simulink model "Laptrinhquydao"  (R2020a)
settings: Solver=VariableStepAuto  StartTime=0.0  StopTime=10.0  RelTol=1e-3
settings Model: Creator=dell  LastModifiedBy=dell

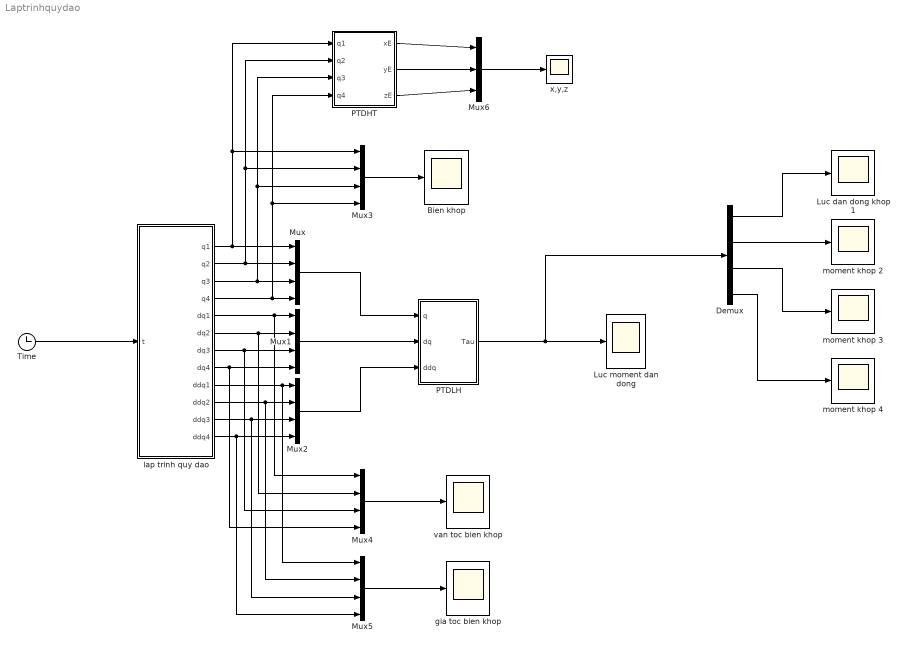
== system Laptrinhquydao ==
  Bien khop : Scope
  Demux : Demux
  "Luc dan dong khop 1 " : Scope
  Luc moment dan dong : Scope
  Mux{,1..5} (6 alike) : Mux
  Mux6 : Mux  Inputs=3
  PTDHT : MATLAB Function  TreatAsAtomicUnit=on
  PTDLH : MATLAB Function  TreatAsAtomicUnit=on
  "Time " : Clock
  gia toc bien khop : Scope
  lap trinh quy dao : MATLAB Function  TreatAsAtomicUnit=on
  moment khop 2 : Scope
  moment khop 3 : Scope
  moment khop 4 : Scope
  "van toc bien khop " : Scope
  x,y,z : Scope
  wires:
  "Time "/1 -> lap trinh quy dao/1(t)
  lap trinh quy dao/1(q1) -> Mux3/1, PTDHT/1(q1), Mux/1
  lap trinh quy dao/2(q2) -> Mux3/2, PTDHT/2(q2), Mux/2
  lap trinh quy dao/3(q3) -> Mux3/3, PTDHT/3(q3), Mux/3
  lap trinh quy dao/4(q4) -> Mux3/4, PTDHT/4(q4), Mux/4
  lap trinh quy dao/5(dq1) -> Mux4/1, Mux1/1
  lap trinh quy dao/6(dq2) -> Mux4/2, Mux1/2
  lap trinh quy dao/7(dq3) -> Mux4/3, Mux1/3
  lap trinh quy dao/8(dq4) -> Mux4/4, Mux1/4
  lap trinh quy dao/9(ddq1) -> Mux5/1, Mux2/1
  lap trinh quy dao/10(ddq2) -> Mux5/2, Mux2/2
  lap trinh quy dao/11(ddq3) -> Mux5/3, Mux2/3
  lap trinh quy dao/12(ddq4) -> Mux5/4, Mux2/4
  Mux1/1 -> PTDLH/2(dq)
  Mux/1 -> PTDLH/1(q)
  Mux2/1 -> PTDLH/3(ddq)
  PTDLH/1(Tau) -> Demux/1, Luc moment dan dong/1
  Mux3/1 -> Bien khop/1
  Mux4/1 -> "van toc bien khop "/1
  Mux5/1 -> gia toc bien khop/1
  Demux/1 -> "Luc dan dong khop 1 "/1
  Demux/2 -> moment khop 2/1
  Demux/3 -> moment khop 3/1
  Demux/4 -> moment khop 4/1
  PTDHT/2(yE) -> Mux6/2
  PTDHT/1(xE) -> Mux6/1
  PTDHT/3(zE) -> Mux6/3
  Mux6/1 -> x,y,z/1

== matlab function Laptrinhquydao/PTDLH ==
  data: q input; Tau output; dq input; ddq input
function Tau = fcn(q,dq,ddq)

[L1, L2, L3, L4,L0,m1,m2,m3,m4,I1x,I1y,I1z,I2x,I2y,I2z,I3x,I3y,I3z,I4x,I4y,I4z]=Parameters();

M=zeros(4,4);
M(1,1)= m1 + m2 + m3 + m4;
M(1,2)= ((-0.3e1 * m4 * L4 * cos(q(4)) - 0.3e1 * L3 * (m3 + 0.2e1 / 0.3e1 * m4)) * cos(q(3)) + 0.3e1 * sin(q(3)) * sin(q(4)) * L4 * m4 - 0.3e1 * L2 * (m2 + 0.2e1 / 0.3e1 * m3 + 0.2e1 / 0.3e1 * m4)) * cos(q(2)) / 0.2e1 + 0.3e1 / 0.2e1 * sin(q(2)) * (sin(q(4)) * L4 * m4 * cos(q(3)) + (m4 * L4 * cos(q(4)) + L3 * (m3 + 0.2e1 / 0.3e1 * m4)) * sin(q(3)));
M(1,3)= ((-0.3e1 * m4 * L4 * cos(q(4)) - 0.3e1 * L3 * (m3 + 0.2e1 / 0.3e1 * m4)) * cos(q(3)) + 0.3e1 * sin(q(3)) * sin(q(4)) * L4 * m4) * cos(q(2)) / 0.2e1 + 0.3e1 / 0.2e1 * sin(q(2)) * (sin(q(4)) * L4 * m4 * cos(q(3)) + (m4 * L4 * cos(q(4)) + L3 * (m3 + 0.2e1 / 0.3e1 * m4)) * sin(q(3)));
M(1,4)= 0.3e1 / 0.2e1 * L4 * ((sin(q(2)) * sin(q(3)) - cos(q(2)) * cos(q(3))) * cos(q(4)) + sin(q(4)) * (cos(q(2)) * sin(q(3)) + sin(q(2)) * cos(q(3)))) * m4;

M(2,1)= ((-0.3e1 * m4 * L4 * cos(q(4)) - 0.3e1 * L3 * (m3 + 0.2e1 / 0.3e1 * m4)) * cos(q(3)) + 0.3e1 * sin(q(3)) * sin(q(4)) * L4 * m4 - 0.3e1 * L2 * (m2 + 0.2e1 / 0.3e1 * m3 + 0.2e1 / 0.3e1 * m4)) * cos(q(2)) / 0.2e1 + 0.3e1 / 0.2e1 * sin(q(2)) * (sin(q(4)) * L4 * m4 * cos(q(3)) + (m4 * L4 * cos(q(4)) + L3 * (m3 + 0.2e1 / 0.3e1 * m4)) * sin(q(3)));
M(2,2)= 0.3e1 * L2 * (m4 * L4 * cos(q(4)) + L3 * (m3 + 0.2e1 / 0.3e1 * m4)) * cos(q(3)) + 0.3e1 * m4 * L4 * L3 * cos(q(4)) - 0.3e1 * m4 * L4 * L2 * sin(q(4)) * sin(q(3)) + ((9 * m2) + 0.4e1 * m3 + 0.4e1 * m4) * L2 ^ 2 / 0.4e1 + (0.4e1 * L3 ^ 2 + 0.9e1 * L4 ^ 2) * m4 / 0.4e1 + 0.9e1 / 0.4e1 * m3 * L3 ^ 2 + I3z + I4z + I2z;
M(2,3)= 0.3e1 / 0.2e1 * L2 * (m4 * L4 * cos(q(4)) + L3 * (m3 + 0.2e1 / 0.3e1 * m4)) * cos(q(3)) + 0.3e1 * m4 * L4 * L3 * cos(q(4)) - 0.3e1 / 0.2e1 * m4 * L4 * L2 * sin(q(4)) * sin(q(3)) + (0.4e1 * L3 ^ 2 + 0.9e1 * L4 ^ 2) * m4 / 0.4e1 + 0.9e1 / 0.4e1 * m3 * L3 ^ 2 + I3z + I4z;
M(2,4)= 0.3e1 / 0.2e1 * m4 * L4 * (L2 * cos(q(3)) + L3) * cos(q(4)) - 0.3e1 / 0.2e1 * m4 * L4 * L2 * sin(q(4)) * sin(q(3)) + 0.9e1 / 0.4e1 * m4 * L4 ^ 2 + I4z;

M(3,1)= ((-0.3e1 * m4 * L4 * cos(q(4)) - 0.3e1 * L3 * (m3 + 0.2e1 / 0.3e1 * m4)) * cos(q(3)) + 0.3e1 * sin(q(3)) * sin(q(4)) * L4 * m4) * cos(q(2)) / 0.2e1 + 0.3e1 / 0.2e1 * sin(q(2)) * (sin(q(4)) * L4 * m4 * cos(q(3)) + (m4 * L4 * cos(q(4)) + L3 * (m3 + 0.2e1 / 0.3e1 * m4)) * sin(q(3)));
M(3,2)= 0.3e1 / 0.2e1 * L2 * (m4 * L4 * cos(q(4)) + L3 * (m3 + 0.2e1 / 0.3e1 * m4)) * cos(q(3)) + 0.3e1 * m4 * L4 * L3 * cos(q(4)) - 0.3e1 / 0.2e1 * m4 * L4 * L2 * sin(q(4)) * sin(q(3)) + (0.4e1 * L3 ^ 2 + 0.9e1 * L4 ^ 2) * m4 / 0.4e1 + 0.9e1 / 0.4e1 * m3 * L3 ^ 2 + I3z + I4z;
M(3,3)= 0.3e1 * m4 * L4 * L3 * cos(q(4)) + ((9 * m3) + 0.4e1 * m4) * L3 ^ 2 / 0.4e1 + 0.9e1 / 0.4e1 * m4 * L4 ^ 2 + I3z + I4z;
M(3,4)= 0.3e1 / 0.2e1 * m4 * L4 * L3 * cos(q(4)) + 0.9e1 / 0.4e1 * m4 * L4 ^ 2 + I4z;

M(4,1)= 0.3e1 / 0.2e1 * L4 * ((sin(q(2)) * sin(q(3)) - cos(q(2)) * cos(q(3))) * cos(q(4)) + sin(q(4)) * (cos(q(2)) * sin(q(3)) + sin(q(2)) * cos(q(3)))) * m4;
M(4,2)= 0.3e1 / 0.2e1 * m4 * L4 * (L2 * cos(q(3)) + L3) * cos(q(4)) - 0.3e1 / 0.2e1 * m4 * L4 * L2 * sin(q(4)) * sin(q(3)) + 0.9e1 / 0.4e1 * m4 * L4 ^ 2 + I4z;
M(4,3)= 0.3e1 / 0.2e1 * m4 * L4 * L3 * cos(q(4)) + 0.9e1 / 0.4e1 * m4 * L4 ^ 2 + I4z;
M(4,4)= 0.9e1 / 0.4e1 * m4 * L4 ^ 2 + I4z;

C=zeros(4,4);

C(1,1)= 0;
C(1,2)= ((0.3e1 * L4 * m4 * (dq(3) + dq(4) + dq(2)) * cos(q(4)) + 0.3e1 * L3 * (dq(3) + dq(2)) * (m3 + 0.2e1 / 0.3e1 * m4)) * cos(q(3)) - 0.3e1 * sin(q(3)) * sin(q(4)) * L4 * m4 * (dq(3) + dq(4) + dq(2)) + 0.3e1 * dq(2) * L2 * (m2 + 0.2e1 / 0.3e1 * m3 + 0.2e1 / 0.3e1 * m4)) * sin(q(2)) / 0.2e1 + 0.3e1 / 0.2e1 * cos(q(2)) * (sin(q(4)) * L4 * m4 * (dq(3) + dq(4) + dq(2)) * cos(q(3)) + sin(q(3)) * (L4 * m4 * (dq(3) + dq(4) + dq(2)) * cos(q(4)) + L3 * (dq(3) + dq(2)) * (m3 + 0.2e1 / 0.3e1 * m4)));
C(1,3)= (0.3e1 * sin(q(4)) * L4 * m4 * (dq(3) + dq(4) + dq(2)) * cos(q(3)) + 0.3e1 * sin(q(3)) * (L4 * m4 * (dq(3) + dq(4) + dq(2)) * cos(q(4)) + L3 * (dq(3) + dq(2)) * (m3 + 0.2e1 / 0.3e1 * m4))) * cos(q(2)) / 0.2e1 + 0.3e1 / 0.2e1 * ((L4 * m4 * (dq(3) + dq(4) + dq(2)) * cos(q(4)) + L3 * (dq(3) + dq(2)) * (m3 + 0.2e1 / 0.3e1 * m4)) * cos(q(3)) - sin(q(3)) * sin(q(4)) * L4 * m4 * (dq(3) + dq(4) + dq(2))) * sin(q(2));
C(1,4)= 0.3e1 / 0.2e1 * L4 * ((cos(q(2)) * sin(q(3)) + sin(q(2)) * cos(q(3))) * cos(q(4)) + (cos(q(2)) * cos(q(3)) - sin(q(2)) * sin(q(3))) * sin(q(4))) * (dq(3) + dq(4) + dq(2)) * m4;

C(2,1)= ((0.3e1 * L4 * m4 * (dq(3) + dq(4) + dq(2)) * cos(q(4)) + 0.3e1 * L3 * (m3 + 0.2e1 / 0.3e1 * m4) * (dq(3) + dq(2))) * cos(q(3)) - 0.3e1 * sin(q(3)) * sin(q(4)) * L4 * m4 * (dq(3) + dq(4) + dq(2)) + 0.3e1 * dq(2) * L2 * (m2 + 0.2e1 / 0.3e1 * m3 + 0.2e1 / 0.3e1 * m4)) * sin(q(2)) / 0.4e1 + 0.3e1 / 0.4e1 * cos(q(2)) * (sin(q(4)) * L4 * m4 * (dq(3) + dq(4) + dq(2)) * cos(q(3)) + sin(q(3)) * (L4 * m4 * (dq(3) + dq(4) + dq(2)) * cos(q(4)) + L3 * (m3 + 0.2e1 / 0.3e1 * m4) * (dq(3) + dq(2))));
C(2,2)= (0.3e1 * sin(q(2)) * sin(q(4)) * L4 * m4 * dq(1) - 0.3e1 * (m4 * L4 * cos(q(4)) + L3 * (m3 + 0.2e1 / 0.3e1 * m4)) * dq(1) * cos(q(2)) - 0.12e2 * (L4 * m4 * (dq(4) + dq(3)) * cos(q(4)) + dq(3) * L3 * (m3 + 0.2e1 / 0.3e1 * m4)) * L2) * sin(q(3)) / 0.4e1 - 0.3e1 / 0.4e1 * dq(1) * ((m4 * L4 * cos(q(4)) + L3 * (m3 + 0.2e1 / 0.3e1 * m4)) * cos(q(3)) + L2 * (m2 + 0.2e1 / 0.3e1 * m3 + 0.2e1 / 0.3e1 * m4)) * sin(q(2)) - 0.3e1 * m4 * ((cos(q(2)) * dq(1) / 0.4e1 + L2 * (dq(4) + dq(3))) * cos(q(3)) + dq(4) * L3) * sin(q(4)) * L4;
C(2,3)= (0.3e1 * sin(q(2)) * sin(q(4)) * L4 * m4 * dq(1) - 0.3e1 * (m4 * L4 * cos(q(4)) + L3 * (m3 + 0.2e1 / 0.3e1 * m4)) * dq(1) * cos(q(2)) - 0.6e1 * (L4 * m4 * (dq(4) + dq(3)) * cos(q(4)) + dq(3) * L3 * (m3 + 0.2e1 / 0.3e1 * m4)) * L2) * sin(q(3)) / 0.4e1 + (-0.6e1 * L4 * m4 * (cos(q(2)) * dq(1) / 0.2e1 + L2 * (dq(4) + dq(3))) * sin(q(4)) - 0.3e1 * (m4 * L4 * cos(q(4)) + L3 * (m3 + 0.2e1 / 0.3e1 * m4)) * dq(1) * sin(q(2))) * cos(q(3)) / 0.4e1 - 0.3e1 * m4 * L4 * L3 * sin(q(4)) * dq(4);
C(2,4)= -0.3e1 / 0.2e1 * (((cos(q(2)) * dq(1) / 0.2e1 + L2 * (dq(4) + dq(3))) * cos(q(3)) - sin(q(2)) * sin(q(3)) * dq(1) / 0.2e1 + dq(4) * L3) * sin(q(4)) + (sin(q(2)) * dq(1) * cos(q(3)) / 0.2e1 + sin(q(3)) * (cos(q(2)) * dq(1) / 0.2e1 + L2 * (dq(4) + dq(3)))) * cos(q(4))) * L4 * m4;

C(3,1)= (0.3e1 * sin(q(4)) * L4 * m4 * (dq(3) + dq(4) + dq(2)) * cos(q(3)) + 0.3e1 * sin(q(3)) * (L4 * m4 * (dq(3) + dq(4) + dq(2)) * cos(q(4)) + L3 * (m3 + 0.2e1 / 0.3e1 * m4) * (dq(3) + dq(2)))) * cos(q(2)) / 0.4e1 + 0.3e1 / 0.4e1 * sin(q(2)) * ((L4 * m4 * (dq(3) + dq(4) + dq(2)) * cos(q(4)) + L3 * (m3 + 0.2e1 / 0.3e1 * m4) * (dq(3) + dq(2))) * cos(q(3)) - sin(q(3)) * sin(q(4)) * L4 * m4 * (dq(3) + dq(4) + dq(2)));
C(3,2)= (0.3e1 * sin(q(2)) * sin(q(4)) * L4 * m4 * dq(1) + 0.6e1 * L4 * m4 * (-cos(q(2)) * dq(1) / 0.2e1 + L2 * (dq(2) - dq(3) / 0.2e1 - dq(4) / 0.2e1)) * cos(q(4)) + 0.6e1 * (m3 + 0.2e1 / 0.3e1 * m4) * L3 * (-cos(q(2)) * dq(1) / 0.2e1 + L2 * (dq(2) - dq(3) / 0.2e1))) * sin(q(3)) / 0.4e1 + (0.6e1 * L4 * m4 * (-cos(q(2)) * dq(1) / 0.2e1 + L2 * (dq(2) - dq(3) / 0.2e1 - dq(4) / 0.2e1)) * sin(q(4)) - 0.3e1 * (m4 * L4 * cos(q(4)) + L3 * (m3 + 0.2e1 / 0.3e1 * m4)) * dq(1) * sin(q(2))) * cos(q(3)) / 0.4e1 - 0.3e1 * m4 * L4 * L3 * sin(q(4)) * dq(4);
C(3,3)= (-0.3e1 * (m4 * L4 * cos(q(4)) + L3 * (m3 + 0.2e1 / 0.3e1 * m4)) * dq(1) * cos(q(2)) + 0.3e1 * sin(q(2)) * sin(q(4)) * L4 * m4 * dq(1) + 0.3e1 * dq(2) * L2 * (m4 * L4 * cos(q(4)) + L3 * (m3 + 0.2e1 / 0.3e1 * m4))) * sin(q(3)) / 0.4e1 + (-0.3e1 * cos(q(2)) * sin(q(4)) * L4 * m4 * dq(1) - 0.3e1 * (m4 * L4 * cos(q(4)) + L3 * (m3 + 0.2e1 / 0.3e1 * m4)) * dq(1) * sin(q(2)) + 0.3e1 * L2 * dq(2) * sin(q(4)) * L4 * m4) * cos(q(3)) / 0.4e1 - 0.3e1 * m4 * L4 * L3 * sin(q(4)) * dq(4);
C(3,4)= 0.3e1 / 0.4e1 * (((L2 * dq(2) - cos(q(2)) * dq(1)) * cos(q(3)) + sin(q(2)) * sin(q(3)) * dq(1) - (2 * dq(4) * L3)) * sin(q(4)) + cos(q(4)) * (-sin(q(2)) * dq(1) * cos(q(3)) + sin(q(3)) * (L2 * dq(2) - cos(q(2)) * dq(1)))) * L4 * m4;

C(4,1)= 0.3e1 / 0.4e1 * L4 * (dq(3) + dq(4) + dq(2)) * m4 * ((cos(q(2)) * sin(q(3)) + sin(q(2)) * cos(q(3))) * cos(q(4)) + (cos(q(2)) * cos(q(3)) - sin(q(2)) * sin(q(3))) * sin(q(4)));
C(4,2)= -0.3e1 / 0.4e1 * L4 * m4 * (((cos(q(2)) * dq(1) + (L2 * (dq(3) + dq(4) - 2 * dq(2)))) * cos(q(3)) - sin(q(2)) * sin(q(3)) * dq(1) - 0.2e1 * (dq(3) - dq(4) / 0.2e1 + dq(2)) * L3) * sin(q(4)) + (sin(q(2)) * dq(1) * cos(q(3)) + (cos(q(2)) * dq(1) + (L2 * (dq(3) + dq(4) - 2 * dq(2)))) * sin(q(3))) * cos(q(4)));
C(4,3)= 0.3e1 / 0.4e1 * (((L2 * dq(2) - cos(q(2)) * dq(1)) * cos(q(3)) + sin(q(2)) * sin(q(3)) * dq(1) + 0.2e1 * (dq(3) - dq(4) / 0.2e1 + dq(2)) * L3) * sin(q(4)) + cos(q(4)) * (-sin(q(2)) * dq(1) * cos(q(3)) + sin(q(3)) * (L2 * dq(2) - cos(q(2)) * dq(1)))) * L4 * m4;
C(4,4)= 0.3e1 / 0.4e1 * L4 * (((L2 * dq(2) - cos(q(2)) * dq(1)) * cos(q(3)) + sin(q(2)) * sin(q(3)) * dq(1) + L3 * (dq(3) + dq(2))) * sin(q(4)) + cos(q(4)) * (-sin(q(2)) * dq(1) * cos(q(3)) + sin(q(3)) * (L2 * dq(2) - cos(q(2)) * dq(1)))) * m4;

G=zeros(4,1);
G(1,1)=0;
G(2,1)= -((15*m4*L4*cos(q(4)) + 15*L3*(m3 + (2*m4)/3))*cos(q(3)) - 15*sin(q(3))*sin(q(4))*L4*m4 + 15*L2*(m2 + (2*m3)/3 + (2*m4)/3))*sin(q(2)) - 15*m4*L4*cos(q(2))*sin(q(4))*cos(q(3)) - 15*sin(q(3))*(m4*L4*cos(q(4)) + L3*(m3 + (2*m4)/3))*cos(q(2));
G(3,1)= (-(15*m4*L4*cos(q(4)) + 15*L3*(m3 + (2*m4)/3))*sin(q(3)) - 15*sin(q(4))*L4*m4*cos(q(3)))*cos(q(2)) + 15*L4*sin(q(2))*sin(q(4))*sin(q(3))*m4 - 15*cos(q(3))*(m4*L4*cos(q(4)) + L3*(m3 + (2*m4)/3))*sin(q(2));
G(4,1)= (-15*sin(q(4))*L4*m4*cos(q(3)) - 15*sin(q(3))*cos(q(4))*L4*m4)*cos(q(2)) - 15*L4*sin(q(2))*cos(q(4))*cos(q(3))*m4 + 15*L4*sin(q(2))*sin(q(4))*sin(q(3))*m4;

Tau=M*ddq+C*dq+G;

== matlab function Laptrinhquydao/lap trinh quy dao ==
  data: t input; q1 output; q2 output; q3 output; q4 output; dq1 output; dq2 output; dq3 output; dq4 output; ddq1 output; ddq2 output; ddq3 output; ddq4 output
function [q1,q2,q3,q4,dq1,dq2,dq3,dq4,ddq1,ddq2,ddq3,ddq4] = fcn(t)
%khai bao vi tri bien khop
q1=0.2+(0.9/100)*t^2-(0.3/500)*t^3;
q2=pi/3+(pi/200)*t^2-(pi/3000)*t^3;
q3=-pi/6+(3*pi/200)*t^2-(pi/1000)*t^3;
q4=pi/6+(pi/100)*t^2-(pi/1500)*t^3;
%khai bao van toc bien khop
dq1=(1.8/100)*t-(0.9/500)*t^2;
dq2=(pi/100)*t-(pi/1000)*t^2;
dq3=(3*pi/100)*t-(3*pi/1000)*t^2;
dq4=(pi/50)*t-(pi/500)*t^2;
%khai bao gia toc bien khop
ddq1=1.8/100-(1.8/500)*t;
ddq2=pi/100-(pi/500)*t;
ddq3=3*pi/100-(3*pi/500)*t;
ddq4=pi/50-(pi/250)*t;

== matlab function Laptrinhquydao/PTDHT ==
  data: q1 input; xE output; q2 input; q3 input; q4 input; yE output; zE output
function [xE,yE,zE] = fcn(q1,q2,q3,q4)
L1 = 0.1;
L2 = 0.4;
L3 = 0.3;
L4 = 0.3;
xE = 0;
yE = (-sin(q2) * cos(q3) - cos(q2) * sin(q3)) * L4 * cos(q4) + (sin(q2) * sin(q3) - cos(q2) * cos(q3)) * L4 * sin(q4) - sin(q2) * L3 * cos(q3) - cos(q2) * L3 * sin(q3) - L2 * sin(q2);
zE = (cos(q2) * cos(q3) - sin(q2) * sin(q3)) * L4 * cos(q4) + (-sin(q2) * cos(q3) - cos(q2) * sin(q3)) * L4 * sin(q4) + cos(q2) * L3 * cos(q3) - sin(q2) * L3 * sin(q3) + L2 * cos(q2) + L1 + q1;
end
